simulink model "SendSensorDataSerialExample"  (R2015a)
settings: Solver=ode3  SolverMode=SingleTasking  StartTime=0.0  StopTime=10.0  RelTol=1e-3
settings Model: ExtModeTrigDuration=2  Creator=kkhoo  LastModifiedBy=kkhoo
settings OptimizationCC: OptimizeModelRefInitCode=on  LifeSpan=1
settings DebuggingCC: UnderspecifiedInitializationDetection=Classic  MergeDetectMultiDrivingBlocksExec=none
settings HardwareCC: ProdBitPerInt=16  ProdBitPerPointer=8  ProdIntDivRoundTo=Zero  ProdEndianess=LittleEndian  ProdWordSize=8  ProdHWDeviceType=Atmel->AVR
settings RTWCC: SystemTargetFile=realtime.tlc  GenerateMakefile=off  TemplateMakefile=realtime.tmf  Description=Run on Target Hardware  RTWVerbose=off  CustomSource=src/Engduino.h src/engduino_wrappers.cpp
settings ERTTargetCC: CombineOutputUpdateFcns=off  ExtModeTransport=3  ExtModeMexFile=ext_serial_win32_comm_rtt  ExtModeMexArgs=0 1 9600  ERTSrcFileBannerTemplate=realtime_code_template.cgt  ERTHdrFileBannerTemplate=realtime_code_template.cgt  ERTDataSrcFileTemplate=realtime_code_template.cgt  ERTDataHdrFileTemplate=realtime_code_template.cgt  ERTCustomFileTemplate=realtime_file_process.tlc

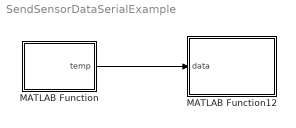
== system SendSensorDataSerialExample ==
  MATLAB Function : MATLAB Function  LoadFcn=|  TreatAsAtomicUnit=on  mask(Thermistor){}
      | set_param(gcs, 'CustomSource', strjoin(unique([strsplit(get_param(gcs, 'CustomSource')) ...
      |  'src/engduino_wrappers.cpp' 'src/Engduino.h'])));
      mask help: Outputs the temperature in milli degrees celsius.
  MATLAB Function12 : MATLAB Function  LoadFcn=|  TreatAsAtomicUnit=on  mask(Thermistor){}
      | set_param(gcs, 'CustomSource', strjoin(unique([strsplit(get_param(gcs, 'CustomSource')) ...
      |  'src/engduino_wrappers.cpp' 'src/Engduino.h'])));
      mask help: Outputs the temperature in milli degrees celsius.
  wires:
  MATLAB Function/1(temp) -> MATLAB Function12/1(data)

== matlab function SendSensorDataSerialExample/MATLAB Function ==
  data: temp output
function temp = thermistor()

temp = 0.0;

if strcmp(coder.target, 'rtw')
    temp = coder.ceval('thermistor_wrapper');
end

== matlab function SendSensorDataSerialExample/MATLAB Function12 ==
  data: data input
function print_serial(data)
if strcmp(coder.target, 'rtw')
    coder.ceval('print_data_serial_wrapper',data);
end
